simulink model "Iniciso3C_Lin"  (R2023a)
settings: Solver=VariableStepAuto  StartTime=0.0  StopTime=20.0  RelTol=1e-3
settings Model: Creator=mezea  LastModifiedBy=Daniela

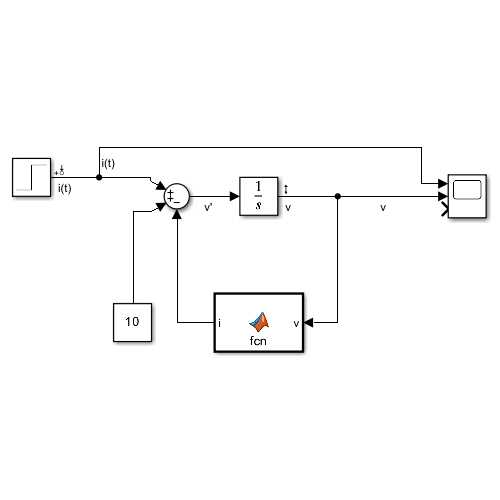
[thumbnail: Simulink's stored preview of the top-level diagram]
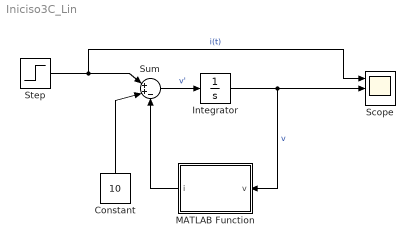
== system Iniciso3C_Lin ==
  Constant : Constant  Value=10
  Integrator : Integrator
  MATLAB Function : MATLAB Function  TreatAsAtomicUnit=on
  Scope : Scope  NumInputPorts=3
  Step : Step  Time=0  SampleTime=0
  Sum : Sum  Inputs=|++-
  wires:
  Integrator/1 -> Scope/2, MATLAB Function/1(v)  "v"
  Sum/1 -> Integrator/1  "v'"
  Step/1 -> Sum/1, Scope/1  "i(t)"
  Constant/1 -> Sum/2
  MATLAB Function/1(i) -> Sum/3

== matlab function Iniciso3C_Lin/MATLAB Function ==
  data: v input; i output
function i = fcn(v)
    i = 5 * exp(0.2 * v);
end
